simulink model "afc_simulation"  (R2019a)
settings: Solver=FixedStepDiscrete  StartTime=0.0  StopTime=50  RelTol=1e-3  EnableMultiTasking=on
values from neighbouring files (symbols this model uses):
  Cbus = 4*P/Vdc_min^2/4/fg    (= 0.0136971290817)    [afc_param.m]
  Cbus_2 = Cbus*2    (= 0.0273942581635)    [afc_param.m]
  Lf_1 = L1    [afc_param.m]
  Lf_2 = L1    [afc_param.m]
  RLf_1 = Lf_1*25    [afc_param.m]
  RLf_2 = Lf_2*25    [afc_param.m]
  Tss = 10e-6    (= 1e-05)    [afc_param.m]
undefined symbols (not defined in the file or in its folder): Ion, Lithium
libraries: simulink x21, powerlib_meascontrol x21, powerlib x17, electricdrivelib x3
(part 1 of 2)
settings Model: Creator=c477  LastModifiedBy=c477
settings SolverCC: AutoInsertRateTranBlk=on
settings OptimizationCC: DefaultParameterBehavior=Inlined  UseDivisionForNetSlopeComputation=on  GainParamInheritBuiltInType=on  UseFloatMulNetSlope=on  InlineInvariantSignals=on  PassReuseOutputArgsAs=Individual arguments  ZeroExternalMemoryAtStartup=off  ZeroInternalMemoryAtStartup=off  NoFixptDivByZeroProtection=on  EfficientFloat2IntCast=on  LifeSpan=1  OptimizeBlockOrder=speed  DifferentSizesBufferReuse=on
settings DebuggingCC: ParameterTunabilityLossMsg=error
settings HardwareCC: ProdLongLongMode=on
settings SFSimCC: MATLABDynamicMemAlloc=off
settings RTWCC: SystemTargetFile=ert.tlc  TemplateMakefile=ert_default_tmf  GenerateReport=on  IncludeHyperlinkInReport=on  LaunchReport=on  TargetLang=C++  GenerateTraceInfo=on  GenerateTraceReport=on  GenerateTraceReportSl=on  GenerateTraceReportSf=on  GenerateTraceReportEml=on
settings CodeAppCC: ForceParamTrailComments=on  IgnoreCustomStorageClasses=off  OperatorAnnotations=on  SimulinkDataObjDesc=on  SFDataObjDesc=on  CustomSymbolStrGlobalVar=rt$N$M  CustomSymbolStrType=$N$M  CustomSymbolStrFcn=$N$M$F  CustomSymbolStrMacro=$N$M  InsertBlockDesc=on
settings ERTTargetCC: TargetLangStandard=C++03 (ISO)  GenerateSampleERTMain=on  IncludeMdlTerminateFcn=off  CombineSignalStateStructs=on  MultiInstanceERTCode=on  CodeInterfacePackaging=C++ class  SupportNonInlinedSFcns=on  InlinedParameterPlacement=NonHierarchical  RootIOFormat=Structure reference  ERTCustomFileTemplate=example_file_process.tlc  ERTFilePackagingFormat=CompactWithDataFile

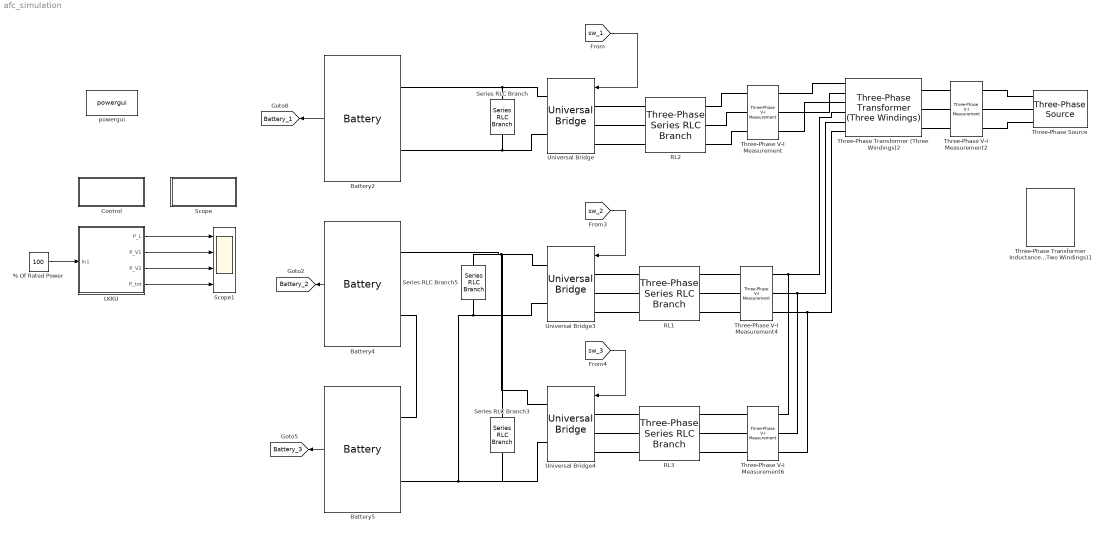
== system afc_simulation ==
  % Of Rated Power : Constant  Value=100
  Battery2 : electricdrivelib/Extra Sources/Battery  BatType=Lithium-Ion  ShowTempParam=off  ThermalPreset="3.3V  2.3Ah  (LiFePO4)"  ShowAgeParam=off  NomV=1000  NomQ=760  SOC=45  Batt_Tr=1  PresetModel=off  MaxQ=760  MinV=818  FullV=1082  Dis_rate=760  R=0.013158  Normal_OP=687.3043  expZone="[1080.3859       37.33913]"  current=[330.4348 330.4348*2 330.4348*5]  Units=Ampere-hour  Tci=20  NomT=25  T2=0  MaxQ2=2.208  FullV2=3.45  Normal_OP2=2.85  expZone2="[3.22       0.015]"  Rca=0.6  ti=1000  Dp=0  Neq0=0  Tsim=1e6  Ta1=25  Qeol=5.4*0.9  Reol=0.013333*1.2  Char_age=[2.3478, 3]  Dis_age=[2.3478, 10]  N1=1500  N2=10500  N3=1000  N4=1400  Ta2=45  N5=950
      settings: SourceProductName=Simscape Electrical
  Battery4 : electricdrivelib/Extra Sources/Battery  BatType=Lithium-Ion  ShowTempParam=off  ThermalPreset="3.3V  2.3Ah  (LiFePO4)"  ShowAgeParam=off  NomV=390  NomQ=641.0256  SOC=45  Batt_Tr=1  PresetModel=on  MaxQ=641.0256  MinV=292.5  FullV=453.955  Dis_rate=278.7068  R=0.006084  Normal_OP=579.7101  expZone="[421.3505      31.49387]"  current=[641.0256 641.0256*2 641.0256*5]  Units=Time  Tci=20  NomT=25  T2=0  MaxQ2=2.208  FullV2=3.45  Normal_OP2=2.85  expZone2="[3.22       0.015]"  Rca=0.6  ti=1000  Dp=0  Neq0=0  Tsim=1e6  Ta1=25  Qeol=5.4*0.9  Reol=0.013333*1.2  Char_age=[2.3478, 3]  Dis_age=[2.3478, 10]  N1=1500  N2=10500  N3=1000  N4=1400  Ta2=45  N5=950
      settings: SourceProductName=Simscape Electrical
  Battery5 : electricdrivelib/Extra Sources/Battery  BatType=Lithium-Ion  ShowTempParam=off  ThermalPreset="3.3V  2.3Ah  (LiFePO4)"  ShowAgeParam=off  NomV=390*2  NomQ=641.0256  SOC=45  Batt_Tr=1  PresetModel=on  MaxQ=641.0256  MinV=585  FullV=907.91  Dis_rate=278.7068  R=0.012168  Normal_OP=579.7101  expZone="[842.701      31.49387]"  current=[641.0256 641.0256*2 641.0256*5]  Units=Time  Tci=20  NomT=25  T2=0  MaxQ2=2.208  FullV2=3.45  Normal_OP2=2.85  expZone2="[3.22       0.015]"  Rca=0.6  ti=1000  Dp=0  Neq0=0  Tsim=1e6  Ta1=25  Qeol=5.4*0.9  Reol=0.013333*1.2  Char_age=[2.3478, 3]  Dis_age=[2.3478, 10]  N1=1500  N2=10500  N3=1000  N4=1400  Ta2=45  N5=950
      settings: SourceProductName=Simscape Electrical
  Control : Subsystem
  LKKU : Subsystem
  RL1 : powerlib/Elements/Three-Phase Series RLC Branch  LConnTagsString=A|B|C  RConnTagsString=A|B|C  BranchType=RL  Resistance=RLf_2  Inductance=Lf_2*1.3  Capacitance=1e-6  Measurements=None
      settings: SourceProductName=Simscape Electrical
  RL2 : powerlib/Elements/Three-Phase Series RLC Branch  LConnTagsString=A|B|C  RConnTagsString=A|B|C  BranchType=RL  Resistance=RLf_1  Inductance=Lf_1  Capacitance=1e-6  Measurements=None
      settings: SourceProductName=Simscape Electrical
  RL3 : powerlib/Elements/Three-Phase Series RLC Branch  LConnTagsString=A|B|C  RConnTagsString=A|B|C  BranchType=RL  Resistance=RLf_2  Inductance=Lf_2*1.3  Capacitance=1e-6  Measurements=None
      settings: SourceProductName=Simscape Electrical
  Scope : Subsystem
  Scope1 : Scope  NumInputPorts=4
  Series RLC Branch : powerlib/Elements/Series RLC Branch  LConnTagsString=__new0  RConnTagsString=__new0  BranchType=C  Resistance=1e-3  Inductance=1e-3  SetiL0=off  InitialCurrent=0  Capacitance=Cbus  Setx0=off  InitialVoltage=0  Measurements=None
      settings: SourceProductName=Simscape Electrical
  Series RLC Branch3 : powerlib/Elements/Series RLC Branch  LConnTagsString=__new0  RConnTagsString=__new0  BranchType=C  Resistance=1e-3  Inductance=1e-3  SetiL0=off  InitialCurrent=0  Capacitance=Cbus_2  Setx0=off  InitialVoltage=0  Measurements=None
      settings: SourceProductName=Simscape Electrical
  Series RLC Branch5 : powerlib/Elements/Series RLC Branch  LConnTagsString=__new0  RConnTagsString=__new0  BranchType=C  Resistance=1e-3  Inductance=1e-3  SetiL0=off  InitialCurrent=0  Capacitance=Cbus_2  Setx0=off  InitialVoltage=0  Measurements=None
      settings: SourceProductName=Simscape Electrical
  Three-Phase Transformer (Three Windings)2 : powerlib/Elements/Three-Phase Transformer (Three Windings)  Winding1Connection=Yg  Winding2Connection=Yg  Winding3Connection=Yg  CoreType=Three single-phase transformers  SetSaturation=off  Hysteresis=off  DataFile='hysteresis'  SetInitialFlux=off  Measurements=None  UNITS=pu  NominalPower=[ 2.5e6 , 60 ]  Winding1=[ 22.8e3, 0, 0]  Winding2=[ 550, 0 , 0]  Winding3=[ 380 , 0 , 0]  Rm=500  Lm=500  L0=0.5  Saturation=[ 0,0 ; 0.0024,1.2 ; 1.0,1.52 ]  InitialFluxes=[0.8 -0.8 0.7]  BreakLoop=on  DiscreteSolver=Trapezoidal iterative  DataType=off  TransfoNumber=1
      settings: SourceProductName=Simscape Electrical  SourceProductBaseCode=PS
  Three-Phase V-I Measurement : powerlib/Measurements/Three-Phase V-I Measurement  VoltageMeasurement=phase-to-ground  SetLabelV=on  LabelV=Vabc_1  Vpu=off  VpuLL=off  CurrentMeasurement=yes  SetLabelI=on  LabelI=Iabc_1  Ipu=off  Pbase=100e6  Vbase=500e3  OutputType=Complex  PhasorSimulation=off  PSBequivalent=0
      settings: SourceProductName=Simscape Electrical
  Three-Phase V-I Measurement2 : powerlib/Measurements/Three-Phase V-I Measurement  VoltageMeasurement=phase-to-ground  SetLabelV=on  LabelV=Vgrid  Vpu=off  VpuLL=off  CurrentMeasurement=yes  SetLabelI=on  LabelI=Igrid  Ipu=off  Pbase=100e6  Vbase=500e3  OutputType=Complex  PhasorSimulation=off  PSBequivalent=0
      settings: SourceProductName=Simscape Electrical
  Three-Phase V-I Measurement4 : powerlib/Measurements/Three-Phase V-I Measurement  VoltageMeasurement=phase-to-ground  SetLabelV=on  LabelV=Vabc_2  Vpu=off  VpuLL=off  CurrentMeasurement=yes  SetLabelI=on  LabelI=Iabc_2  Ipu=off  Pbase=100e6  Vbase=500e3  OutputType=Complex  PhasorSimulation=off  PSBequivalent=0
      settings: SourceProductName=Simscape Electrical
  Three-Phase V-I Measurement6 : powerlib/Measurements/Three-Phase V-I Measurement  VoltageMeasurement=phase-to-ground  SetLabelV=on  LabelV=Vabc_3  Vpu=off  VpuLL=off  CurrentMeasurement=yes  SetLabelI=on  LabelI=Iabc_3  Ipu=off  Pbase=100e6  Vbase=500e3  OutputType=Complex  PhasorSimulation=off  PSBequivalent=0
      settings: SourceProductName=Simscape Electrical
  Three-Phase Source : powerlib/Electrical Sources/Three-Phase Source  InternalConnection=Yg  VoltagePhases=off  Voltage=22.8e3  PhaseAngle=0  Voltage_phases=[25e3 25e3 25e3]/sqrt(3)  PhaseAngles_phases=[0 -120 +120]  Frequency=60  NonIdealSource=off  SpecifyImpedance=off  Resistance=0.8929  Inductance=16.58e-3  ShortCircuitLevel=100e6  BaseVoltage=25e3  XRratio=7  BusType=swing  Pref=10e3  Qref=0  Prefabc=[10e3, 10e3, 10e3]  Qrefabc=[0, 0, 0]  Qmin=-inf  Qmax=inf
      settings: SourceProductName=Simscape Electrical
  Three-Phase Transformer Inductance Matrix Type (Two Windings)1 : powerlib/Elements/Three-Phase Transformer Inductance Matrix Type (Two Windings)  CoreType=Three-limb or five-limb core  Winding1Connection=Yg  Winding2Connection=Yg  AutoTransformer=off  Measurements=None  NominalPower=[1e6, 60]  VLLnom=[22.8e3, 550]  WindingResistances=[0, 0]  NoLoadIexcPos=2  NoLoadPlossPos=1000  ShortCircuitReactancePos=0.06  ShortCircuitReactancePosAuto=0.06  NoLoadIexcZero=100  NoLoadPlossZero=1500  ShortCircuitReactanceZero=0.03  ShortCircuitReactanceZeroAuto=0.03
      settings: SourceProductName=Simscape Electrical  SourceProductBaseCode=PS
  Universal Bridge : powerlib/Power Electronics/Universal Bridge  Arms=3  SnubberResistance=1e5  SnubberCapacitance=inf  Device=IGBT / Diodes  Ron=1e-3  Lon=0  ForwardVoltages="[  0  0  ]"  ForwardVoltage=0  GTOparameters=[ 10e-6 , 20e-6 ]  IGBTparameters=[ 1e-6 , 2e-6 ]  Measurements=None  Measurements_2=None  converterType=Rectifier
      settings: SourceProductName=Simscape Electrical
  Universal Bridge3 : powerlib/Power Electronics/Universal Bridge  Arms=3  SnubberResistance=1e5  SnubberCapacitance=inf  Device=IGBT / Diodes  Ron=1e-3  Lon=0  ForwardVoltages="[  0  0  ]"  ForwardVoltage=0  GTOparameters=[ 10e-6 , 20e-6 ]  IGBTparameters=[ 1e-6 , 2e-6 ]  Measurements=None  Measurements_2=None  converterType=Rectifier
      settings: SourceProductName=Simscape Electrical
  Universal Bridge4 : powerlib/Power Electronics/Universal Bridge  Arms=3  SnubberResistance=1e5  SnubberCapacitance=inf  Device=IGBT / Diodes  Ron=1e-3  Lon=0  ForwardVoltages="[  0  0  ]"  ForwardVoltage=0  GTOparameters=[ 10e-6 , 20e-6 ]  IGBTparameters=[ 1e-6 , 2e-6 ]  Measurements=None  Measurements_2=None  converterType=Rectifier
      settings: SourceProductName=Simscape Electrical
  powergui : powerlib/powergui  Priority=1  SimulationMode=Discrete  SampleTime=Tss  frequency=60  Iterations=50  frequencyindice=0  Pbase=100e6  ErrMax=1e-4  UnitsV=kV  UnitsW=MW  buscounter=0  FunctionMessages=off  echomessages=off  EnableUseOfTLC=off  CurrentSourceSwitches=off  DisableSnubberDevices=off  DisableRonSwitches=off  DisableVfSwitches=off  DisplayEquations=off  AutomaticDiscreteSolvers=off  SolverType=Tustin/Backward Euler (TBE)  Interpol=off  ExternalGateDelay=off  methode=off  Ts=100  x0status=blocks  SPID=on  SwTol=0  HookPort=off  NonlinearTolerance=0  nMaxIteration=15  ContinueOnMaxIteration=off  RestoreLinks=warning  ResistiveCurrentMeasurement=off  Frange=[0:2:500]  Ylog=off  Xlog=on  ShowGrid=off  save=off  variable=ZData  structure=0  ZoomFFT=off  StartTime=0.0  cycles=1  DisplayStyle=1  fundamental=60  FreqAxis=off  MaxFrequency=1000  frequencyindicesteady=1  RmsSteady=1  display=off
      settings: SourceProductName=Simscape Electrical
  tag scope: Battery_1=global, Battery_2=global, Battery_3=global
  wires:
  Battery2/1 -> [Battery_1]
  [sw_1] -> Universal Bridge/1
  [sw_2] -> Universal Bridge3/1
  Battery4/1 -> [Battery_2]
  Battery5/1 -> [Battery_3]
  [sw_3] -> Universal Bridge4/1
  % Of Rated Power/1 -> LKKU/1(In1)
  LKKU/1(P_L) -> Scope1/1
  LKKU/2(P_V1) -> Scope1/2
  LKKU/3(P_V2) -> Scope1/3
  LKKU/4(P_tot) -> Scope1/4
  connections:
  RL2/LConn2 -- Universal Bridge/LConn2
  RL2/LConn1 -- Universal Bridge/LConn1
  RL2/LConn3 -- Universal Bridge/LConn3
  Universal Bridge/RConn2 -- Series RLC Branch/RConn1 -- Battery2/LConn2
  Universal Bridge/RConn1 -- Series RLC Branch/LConn1 -- Battery2/LConn1
  Three-Phase Source/RConn1 -- Three-Phase V-I Measurement2/LConn1
  Three-Phase V-I Measurement2/LConn2 -- Three-Phase Source/RConn2
  Three-Phase V-I Measurement2/LConn3 -- Three-Phase Source/RConn3
  Three-Phase V-I Measurement/LConn3 -- RL2/RConn3
  Three-Phase V-I Measurement/LConn1 -- RL2/RConn1
  Three-Phase V-I Measurement/LConn2 -- RL2/RConn2
  Three-Phase V-I Measurement6/RConn1 -- Three-Phase V-I Measurement4/RConn1 -- Three-Phase Transformer (Three Windings)2/RConn4
  Three-Phase V-I Measurement6/RConn2 -- Three-Phase Transformer (Three Windings)2/RConn5 -- Three-Phase V-I Measurement4/RConn2
  Three-Phase V-I Measurement6/RConn3 -- Three-Phase Transformer (Three Windings)2/RConn6 -- Three-Phase V-I Measurement4/RConn3
  Battery4/LConn2 -- Battery5/LConn1
  RL1/LConn1 -- Universal Bridge3/LConn1
  RL1/LConn2 -- Universal Bridge3/LConn2
  RL1/LConn3 -- Universal Bridge3/LConn3
  RL1/RConn2 -- Three-Phase V-I Measurement4/LConn2
  RL1/RConn1 -- Three-Phase V-I Measurement4/LConn1
  RL1/RConn3 -- Three-Phase V-I Measurement4/LConn3
  Universal Bridge3/RConn1 -- Series RLC Branch5/LConn1 -- Battery4/LConn1 -- Universal Bridge4/RConn1 -- Series RLC Branch3/LConn1
  RL3/RConn1 -- Three-Phase V-I Measurement6/LConn1
  RL3/LConn3 -- Universal Bridge4/LConn3
  RL3/LConn2 -- Universal Bridge4/LConn2
  RL3/LConn1 -- Universal Bridge4/LConn1
  RL3/RConn2 -- Three-Phase V-I Measurement6/LConn2
  RL3/RConn3 -- Three-Phase V-I Measurement6/LConn3
  Series RLC Branch5/RConn1 -- Universal Bridge3/RConn2 -- Universal Bridge4/RConn2 -- Series RLC Branch3/RConn1 -- Battery5/LConn2
  Three-Phase Transformer (Three Windings)2/LConn1 -- Three-Phase V-I Measurement2/RConn1
  Three-Phase Transformer (Three Windings)2/LConn2 -- Three-Phase V-I Measurement2/RConn2
  Three-Phase Transformer (Three Windings)2/LConn3 -- Three-Phase V-I Measurement2/RConn3
  Three-Phase Transformer (Three Windings)2/RConn1 -- Three-Phase V-I Measurement/RConn1
  Three-Phase Transformer (Three Windings)2/RConn2 -- Three-Phase V-I Measurement/RConn2
  Three-Phase Transformer (Three Windings)2/RConn3 -- Three-Phase V-I Measurement/RConn3

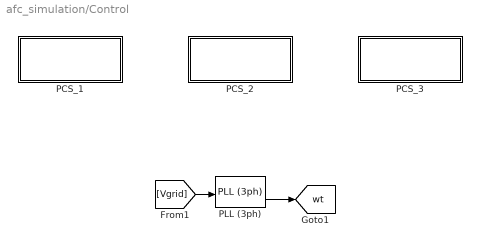
== system afc_simulation/Control ==
  PCS_1 : Subsystem
  PCS_2 : Subsystem
  PCS_3 : Subsystem
  PLL (3ph) : powerlib_meascontrol/PLL/PLL (3ph)  Fmin=45  Par_Init=[0, 50]  ParK=[180, 3200, 1]  TcD=1e-4  MaxRateChangeFreq=12  FilterCutOffFreq=25  Ts=Tss  AGC=on
      settings: SourceProductName=Simscape Electrical
  tag scope: wt=global
  wires:
  [Vgrid] -> PLL (3ph)/1
  PLL (3ph)/2 -> [wt]

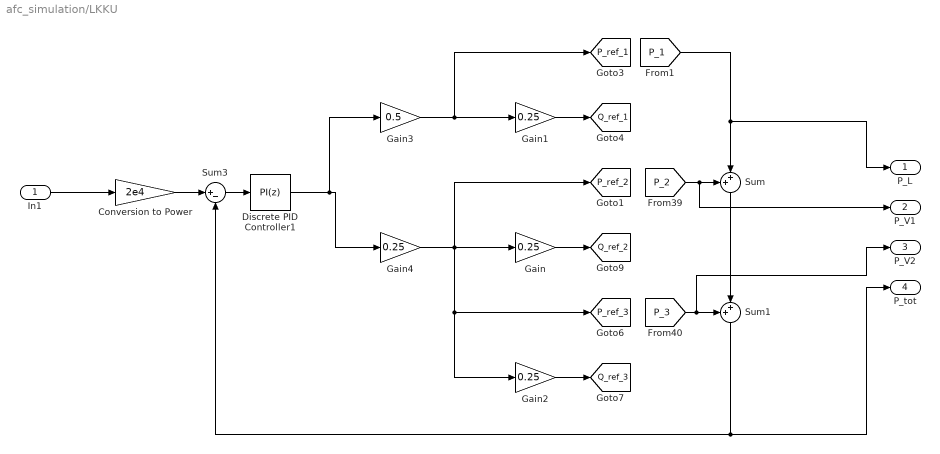
== system afc_simulation/LKKU ==
  In1 : Inport
  Conversion to Power : Gain  Gain=2e4
  Discrete PID Controller1 : simulink/Continuous/PID Controller  Controller=PI  Form=Parallel  TimeDomain=Discrete-time  SampleTime=Tss*30  IntegratorMethod=Forward Euler  FilterMethod=Forward Euler  ControllerParametersSource=internal  P=30  I=60  D=0.5  UseFilter=on  N=100  TunerSelectOption=Transfer Function Based (PID Tuner App)  InitialConditionSource=internal  InitialConditionForIntegrator=0  InitialConditionForFilter=0  DifferentiatorICPrevScaledInput=0  ExternalReset=none  TrackingMode=off  Kt=1  LimitOutput=off  UpperSaturationLimit=inf  LowerSaturationLimit=-inf  LinearizeAsGain=off  AntiWindupMode=none  Kb=1  POutMin=[]  POutMax=[]  IOutMin=[]  IOutMax=[]  DOutMin=[]  DOutMax=[]  NOutMin=[]  NOutMax=[]  SumOutMin=[]  SumOutMax=[]  SaturationOutMin=[]  SaturationOutMax=[]  PParamMin=[]  PParamMax=[]  IParamMin=[]  IParamMax=[]  DParamMin=[]  DParamMax=[]  NParamMin=[]  NParamMax=[]  KbParamMin=[]  KbParamMax=[]  KtParamMin=[]  KtParamMax=[]  KbOutMin=[]  KbOutMax=[]  KtOutMin=[]  KtOutMax=[]  IntegratorOutMin=[]  IntegratorOutMax=[]  FilterOutMin=[]  FilterOutMax=[]  SumI1OutMin=[]  SumI1OutMax=[]  SumI2OutMin=[]  SumI2OutMax=[]  SumI3OutMin=[]  SumI3OutMax=[]  SumI4OutMin=[]  SumI4OutMax=[]  SumDOutMin=[]  SumDOutMax=[]  DifferentiatorOutMin=[]  DifferentiatorOutMax=[]  FilterDiffOutCoefMin=[]  FilterDiffOutCoefMax=[]  ReciprocalOutMin=[]  ReciprocalOutMax=[]  SumDenOutMin=[]  SumDenOutMax=[]  SumNumOutMin=[]  SumNumOutMax=[]  DivideOutMin=[]  DivideOutMax=[]  IntegratorContinuousStateAttributes=''  IntegratorStateMustResolveToSignalObject=off  IntegratorRTWStateStorageClass=Auto  FilterContinuousStateAttributes=''  FilterStateMustResolveToSignalObject=off  FilterRTWStateStorageClass=Auto  ParallelPVariant=InternalParameters  IdealPVariant=Disabled  IVariant=InternalParameters  DVariant=Disabled  IntegratorVariant=Discrete  SatVariant=Disabled  AWVariant=Passthrough  PCopyVariant=Disabled  TRVariant=Disabled  FdbkBlocksVariant=Forward  IdealPFdbkVariant=Disabled  SatFdbkVariant=Disabled  DerivativeFilterVariant=Disabled  NVariant=Disabled  NCopyVariant=Disabled_SignalSpec  FilterICVariant=Disabled  IntegratorICVariant=InternalICs  ExternalResetVariant=Disabled  TRSumVariant=Passthrough  SumFdbkVariant=Disabled  SumVariant=Sum_PI
  Gain{,1..2,4} (4 alike) : Gain  Gain=0.25
  Gain3 : Gain  Gain=0.5
  Sum : Sum  Inputs=++|
  Sum1 : Sum  Inputs=++|
  Sum3 : Sum  Inputs=|+-
  P_L : Outport
  P_V1 : Outport  Port=2
  P_V2 : Outport  Port=3
  P_tot : Outport  Port=4
  tag scope: P_ref_1=global, P_ref_2=global, P_ref_3=global, Q_ref_1=global, Q_ref_2=global, Q_ref_3=global
  wires:
  Sum1/1 -> P_tot/1, Sum3/2
  In1/1 -> Conversion to Power/1
  [P_2] -> P_V1/1, Sum/1
  Discrete PID Controller1/1 -> Gain3/1, Gain4/1
  [P_3] -> P_V2/1, Sum1/1
  Conversion to Power/1 -> Sum3/1
  Gain4/1 -> [P_ref_3], Gain2/1, [P_ref_2], Gain/1
  Sum3/1 -> Discrete PID Controller1/1
  Sum/1 -> Sum1/2
  Gain1/1 -> [Q_ref_1]
  Gain2/1 -> [Q_ref_3]
  [P_1] -> P_L/1, Sum/2
  Gain3/1 -> [P_ref_1], Gain1/1
  Gain/1 -> [Q_ref_2]

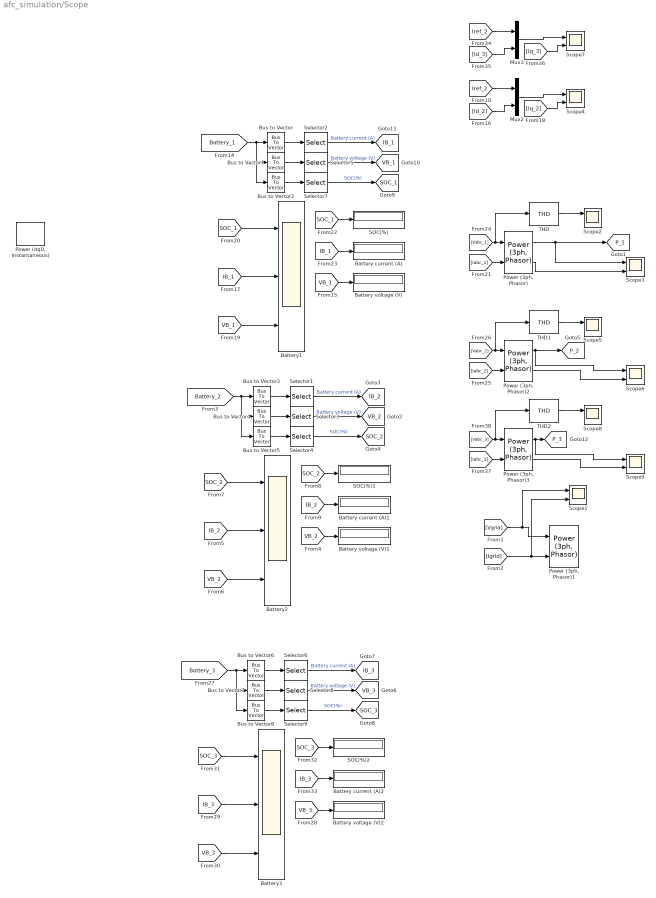
== system afc_simulation/Scope ==
  Battery current (A) : Display
  Battery current (A)1 : Display
  Battery current (A)2 : Display
  Battery voltage (V) : Display
  Battery voltage (V)1 : Display
  Battery voltage (V)2 : Display
  Battery1 : Scope  NumInputPorts=3
  Battery2 : Scope  NumInputPorts=3
  Battery3 : Scope  NumInputPorts=3
  Bus to Vector{,1..8} (9 alike) : BusToVector
  Mux2 : Mux  Inputs=2
  Mux3 : Mux  Inputs=2
  Power (3ph, Phasor){,1..3} (4 alike) : powerlib_meascontrol/Measurements/Power (3ph, Phasor)
      settings: SourceProductName=Simscape Electrical  SourceProductBaseCode=PS
  "Power (dq0, Instantaneous)" : powerlib_meascontrol/Measurements/Power (dq0, Instantaneous)
      settings: SourceProductName=Simscape Electrical  SourceProductBaseCode=PS
  SOC(%) : Display
  SOC(%)1 : Display
  SOC(%)2 : Display
  Scope{1..9} (9 alike) : Scope  NumInputPorts=2
  Selector1 : Selector  InputPortWidth=3  IndexOptions=Index vector (dialog)  Indices=[2]  OutputSizes=1
  Selector2 : Selector  InputPortWidth=3  IndexOptions=Index vector (dialog)  Indices=[2]  OutputSizes=1
  Selector3 : Selector  InputPortWidth=3  IndexOptions=Index vector (dialog)  Indices=[3]  OutputSizes=1
  Selector4 : Selector  InputPortWidth=3  IndexOptions=Index vector (dialog)  Indices=[1]  OutputSizes=1
  Selector5 : Selector  InputPortWidth=3  IndexOptions=Index vector (dialog)  Indices=[3]  OutputSizes=1
  Selector6 : Selector  InputPortWidth=3  IndexOptions=Index vector (dialog)  Indices=[2]  OutputSizes=1
  Selector7 : Selector  InputPortWidth=3  IndexOptions=Index vector (dialog)  Indices=[1]  OutputSizes=1
  Selector8 : Selector  InputPortWidth=3  IndexOptions=Index vector (dialog)  Indices=[3]  OutputSizes=1
  Selector9 : Selector  InputPortWidth=3  IndexOptions=Index vector (dialog)  Indices=[1]  OutputSizes=1
  THD : powerlib_meascontrol/Measurements/THD  Freq=60  Ts=Tss
      settings: SourceProductName=Simscape Electrical
  THD1 : powerlib_meascontrol/Measurements/THD  Freq=60  Ts=Tss
      settings: SourceProductName=Simscape Electrical
  THD2 : powerlib_meascontrol/Measurements/THD  Freq=60  Ts=Tss
      settings: SourceProductName=Simscape Electrical
  tag scope: IB_1=global, IB_2=global, IB_3=global, P_1=global, P_2=global, P_3=global, SOC_1=global, SOC_2=global, SOC_3=global, VB_1=global, VB_2=global, VB_3=global
  wires:
  [IB_1] -> Battery current (A)/1
  Selector7/1 -> [SOC_1]  "SOC(%)"
  Bus to Vector1/1 -> Selector5/1
  [VB_1] -> Battery1/3
  [VB_1] -> Battery voltage (V)/1
  [SOC_1] -> Battery1/1
  [SOC_1] -> SOC(%)/1
  Selector2/1 -> [IB_1]  "Battery current (A)"
  Bus to Vector/1 -> Selector2/1
  [IB_1] -> Battery1/2
  Selector5/1 -> [VB_1]  "Battery voltage (V)"
  Bus to Vector2/1 -> Selector7/1
  [Battery_1] -> Bus to Vector/1, Bus to Vector1/1, Bus to Vector2/1
  [Vabc_1] -> THD/1, "Power (3ph, Phasor)"/1
  [Iabc_1] -> "Power (3ph, Phasor)"/2
  "Power (3ph, Phasor)"/2 -> Scope3/2
  [Vgrid] -> Scope1/1, "Power (3ph, Phasor)1"/1
  [Igrid] -> Scope1/2, "Power (3ph, Phasor)1"/2
  THD/1 -> Scope2/1
  [Battery_2] -> Bus to Vector5/1, Bus to Vector4/1, Bus to Vector3/1
  Bus to Vector5/1 -> Selector4/1
  Selector3/1 -> [VB_2]  "Battery voltage (V)"
  [IB_2] -> Battery2/2
  Bus to Vector3/1 -> Selector1/1
  Selector1/1 -> [IB_2]  "Battery current (A)"
  [SOC_2] -> SOC(%)1/1
  [SOC_2] -> Battery2/1
  [VB_2] -> Battery voltage (V)1/1
  [VB_2] -> Battery2/3
  Bus to Vector4/1 -> Selector3/1
  Selector4/1 -> [SOC_2]  "SOC(%)"
  [IB_2] -> Battery current (A)1/1
  [Iref_2] -> Mux2/1
  [Iq_2] -> Scope4/2
  Mux2/1 -> Scope4/1
  [Id_2] -> Mux2/2
  THD1/1 -> Scope5/1
  "Power (3ph, Phasor)2"/1 -> [P_2], Scope6/1
  "Power (3ph, Phasor)2"/2 -> Scope6/2
  [Iabc_2] -> "Power (3ph, Phasor)2"/2
  [Vabc_2] -> "Power (3ph, Phasor)2"/1, THD1/1
  [IB_3] -> Battery current (A)2/1
  Selector9/1 -> [SOC_3]  "SOC(%)"
  Bus to Vector7/1 -> Selector8/1
  [VB_3] -> Battery3/3
  [VB_3] -> Battery voltage (V)2/1
  [SOC_3] -> Battery3/1
  [SOC_3] -> SOC(%)2/1
  Selector6/1 -> [IB_3]  "Battery current (A)"
  Bus to Vector6/1 -> Selector6/1
  [IB_3] -> Battery3/2
  Selector8/1 -> [VB_3]  "Battery voltage (V)"
  Bus to Vector8/1 -> Selector9/1
  [Battery_3] -> Bus to Vector6/1, Bus to Vector7/1, Bus to Vector8/1
  [Id_3] -> Mux3/2
  Mux3/1 -> Scope7/1
  [Iq_3] -> Scope7/2
  [Iref_2] -> Mux3/1
  [Vabc_3] -> THD2/1, "Power (3ph, Phasor)3"/1
  [Iabc_3] -> "Power (3ph, Phasor)3"/2
  "Power (3ph, Phasor)3"/2 -> Scope9/2
  "Power (3ph, Phasor)3"/1 -> Scope9/1, [P_3]
  THD2/1 -> Scope8/1
  "Power (3ph, Phasor)"/1 -> [P_1], Scope3/1

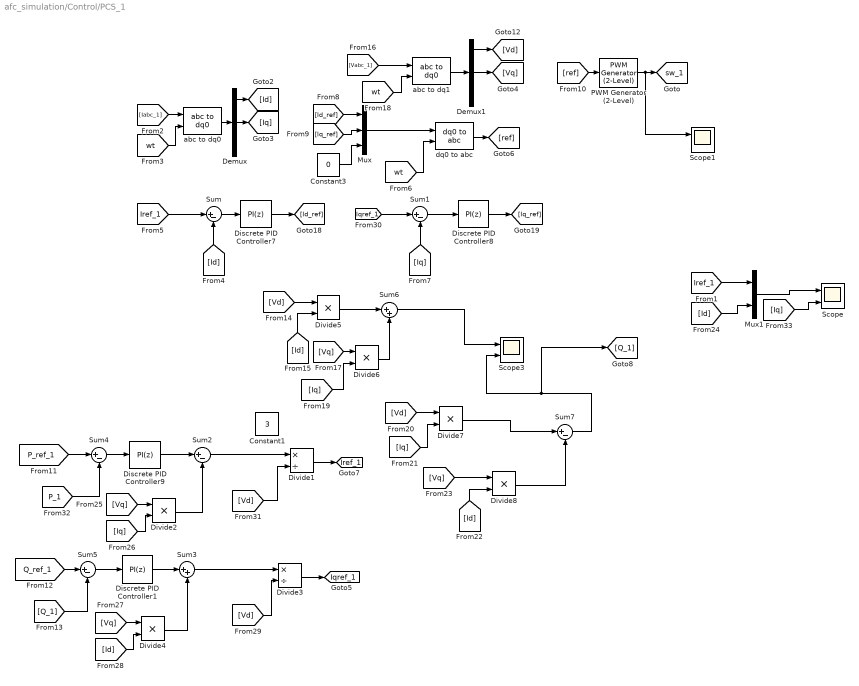
== system afc_simulation/Control/PCS_1 ==
  Constant1 : Constant  Value=3
  Constant3 : Constant  Value=0
  Demux : Demux  Outputs=3
  Demux1 : Demux  Outputs=3
  Discrete PID Controller1 : simulink/Continuous/PID Controller  Controller=PI  Form=Parallel  TimeDomain=Discrete-time  SampleTime=Tss  IntegratorMethod=Forward Euler  FilterMethod=Forward Euler  ControllerParametersSource=internal  P=0.001  I=10  D=0.0001  UseFilter=on  N=100  TunerSelectOption=Transfer Function Based (PID Tuner App)  InitialConditionSource=internal  InitialConditionForIntegrator=0  InitialConditionForFilter=0  DifferentiatorICPrevScaledInput=0  ExternalReset=none  TrackingMode=off  Kt=1  LimitOutput=off  UpperSaturationLimit=1.2  LowerSaturationLimit=0  LinearizeAsGain=off  AntiWindupMode=none  Kb=1  POutMin=[]  POutMax=[]  IOutMin=[]  IOutMax=[]  DOutMin=[]  DOutMax=[]  NOutMin=[]  NOutMax=[]  SumOutMin=[]  SumOutMax=[]  SaturationOutMin=[]  SaturationOutMax=[]  PParamMin=[]  PParamMax=[]  IParamMin=[]  IParamMax=[]  DParamMin=[]  DParamMax=[]  NParamMin=[]  NParamMax=[]  KbParamMin=[]  KbParamMax=[]  KtParamMin=[]  KtParamMax=[]  KbOutMin=[]  KbOutMax=[]  KtOutMin=[]  KtOutMax=[]  IntegratorOutMin=[]  IntegratorOutMax=[]  FilterOutMin=[]  FilterOutMax=[]  SumI1OutMin=[]  SumI1OutMax=[]  SumI2OutMin=[]  SumI2OutMax=[]  SumI3OutMin=[]  SumI3OutMax=[]  SumI4OutMin=[]  SumI4OutMax=[]  SumDOutMin=[]  SumDOutMax=[]  DifferentiatorOutMin=[]  DifferentiatorOutMax=[]  FilterDiffOutCoefMin=[]  FilterDiffOutCoefMax=[]  ReciprocalOutMin=[]  ReciprocalOutMax=[]  SumDenOutMin=[]  SumDenOutMax=[]  SumNumOutMin=[]  SumNumOutMax=[]  DivideOutMin=[]  DivideOutMax=[]  IntegratorContinuousStateAttributes=''  IntegratorStateMustResolveToSignalObject=off  IntegratorRTWStateStorageClass=Auto  FilterContinuousStateAttributes=''  FilterStateMustResolveToSignalObject=off  FilterRTWStateStorageClass=Auto  ParallelPVariant=InternalParameters  IdealPVariant=Disabled  IVariant=InternalParameters  DVariant=Disabled  IntegratorVariant=Discrete  SatVariant=Disabled  AWVariant=Passthrough  PCopyVariant=Disabled  TRVariant=Disabled  FdbkBlocksVariant=Forward  IdealPFdbkVariant=Disabled  SatFdbkVariant=Disabled  DerivativeFilterVariant=Disabled  NVariant=Disabled  NCopyVariant=Disabled_SignalSpec  FilterICVariant=Disabled  IntegratorICVariant=InternalICs  ExternalResetVariant=Disabled  TRSumVariant=Passthrough  SumFdbkVariant=Disabled  SumVariant=Sum_PI
  Discrete PID Controller7 : simulink/Continuous/PID Controller  Controller=PI  Form=Parallel  TimeDomain=Discrete-time  SampleTime=Tss  IntegratorMethod=Forward Euler  FilterMethod=Forward Euler  ControllerParametersSource=internal  P=2  I=3  D=0  UseFilter=on  N=100  TunerSelectOption=Transfer Function Based (PID Tuner App)  InitialConditionSource=internal  InitialConditionForIntegrator=0  InitialConditionForFilter=0  DifferentiatorICPrevScaledInput=0  ExternalReset=none  TrackingMode=off  Kt=1  LimitOutput=off  UpperSaturationLimit=1.2  LowerSaturationLimit=0  LinearizeAsGain=off  AntiWindupMode=none  Kb=1  POutMin=[]  POutMax=[]  IOutMin=[]  IOutMax=[]  DOutMin=[]  DOutMax=[]  NOutMin=[]  NOutMax=[]  SumOutMin=[]  SumOutMax=[]  SaturationOutMin=[]  SaturationOutMax=[]  PParamMin=[]  PParamMax=[]  IParamMin=[]  IParamMax=[]  DParamMin=[]  DParamMax=[]  NParamMin=[]  NParamMax=[]  KbParamMin=[]  KbParamMax=[]  KtParamMin=[]  KtParamMax=[]  KbOutMin=[]  KbOutMax=[]  KtOutMin=[]  KtOutMax=[]  IntegratorOutMin=[]  IntegratorOutMax=[]  FilterOutMin=[]  FilterOutMax=[]  SumI1OutMin=[]  SumI1OutMax=[]  SumI2OutMin=[]  SumI2OutMax=[]  SumI3OutMin=[]  SumI3OutMax=[]  SumI4OutMin=[]  SumI4OutMax=[]  SumDOutMin=[]  SumDOutMax=[]  DifferentiatorOutMin=[]  DifferentiatorOutMax=[]  FilterDiffOutCoefMin=[]  FilterDiffOutCoefMax=[]  ReciprocalOutMin=[]  ReciprocalOutMax=[]  SumDenOutMin=[]  SumDenOutMax=[]  SumNumOutMin=[]  SumNumOutMax=[]  DivideOutMin=[]  DivideOutMax=[]  IntegratorContinuousStateAttributes=''  IntegratorStateMustResolveToSignalObject=off  IntegratorRTWStateStorageClass=Auto  FilterContinuousStateAttributes=''  FilterStateMustResolveToSignalObject=off  FilterRTWStateStorageClass=Auto  ParallelPVariant=InternalParameters  IdealPVariant=Disabled  IVariant=InternalParameters  DVariant=Disabled  IntegratorVariant=Discrete  SatVariant=Disabled  AWVariant=Passthrough  PCopyVariant=Disabled  TRVariant=Disabled  FdbkBlocksVariant=Forward  IdealPFdbkVariant=Disabled  SatFdbkVariant=Disabled  DerivativeFilterVariant=Disabled  NVariant=Disabled  NCopyVariant=Disabled_SignalSpec  FilterICVariant=Disabled  IntegratorICVariant=InternalICs  ExternalResetVariant=Disabled  TRSumVariant=Passthrough  SumFdbkVariant=Disabled  SumVariant=Sum_PI
  Discrete PID Controller8 : simulink/Continuous/PID Controller  Controller=PI  Form=Parallel  TimeDomain=Discrete-time  SampleTime=Tss  IntegratorMethod=Forward Euler  FilterMethod=Forward Euler  ControllerParametersSource=internal  P=2  I=3  D=0  UseFilter=on  N=100  TunerSelectOption=Transfer Function Based (PID Tuner App)  InitialConditionSource=internal  InitialConditionForIntegrator=0  InitialConditionForFilter=0  DifferentiatorICPrevScaledInput=0  ExternalReset=none  TrackingMode=off  Kt=1  LimitOutput=off  UpperSaturationLimit=1.1  LowerSaturationLimit=-1.1  LinearizeAsGain=off  AntiWindupMode=none  Kb=1  POutMin=[]  POutMax=[]  IOutMin=[]  IOutMax=[]  DOutMin=[]  DOutMax=[]  NOutMin=[]  NOutMax=[]  SumOutMin=[]  SumOutMax=[]  SaturationOutMin=[]  SaturationOutMax=[]  PParamMin=[]  PParamMax=[]  IParamMin=[]  IParamMax=[]  DParamMin=[]  DParamMax=[]  NParamMin=[]  NParamMax=[]  KbParamMin=[]  KbParamMax=[]  KtParamMin=[]  KtParamMax=[]  KbOutMin=[]  KbOutMax=[]  KtOutMin=[]  KtOutMax=[]  IntegratorOutMin=[]  IntegratorOutMax=[]  FilterOutMin=[]  FilterOutMax=[]  SumI1OutMin=[]  SumI1OutMax=[]  SumI2OutMin=[]  SumI2OutMax=[]  SumI3OutMin=[]  SumI3OutMax=[]  SumI4OutMin=[]  SumI4OutMax=[]  SumDOutMin=[]  SumDOutMax=[]  DifferentiatorOutMin=[]  DifferentiatorOutMax=[]  FilterDiffOutCoefMin=[]  FilterDiffOutCoefMax=[]  ReciprocalOutMin=[]  ReciprocalOutMax=[]  SumDenOutMin=[]  SumDenOutMax=[]  SumNumOutMin=[]  SumNumOutMax=[]  DivideOutMin=[]  DivideOutMax=[]  IntegratorContinuousStateAttributes=''  IntegratorStateMustResolveToSignalObject=off  IntegratorRTWStateStorageClass=Auto  FilterContinuousStateAttributes=''  FilterStateMustResolveToSignalObject=off  FilterRTWStateStorageClass=Auto  ParallelPVariant=InternalParameters  IdealPVariant=Disabled  IVariant=InternalParameters  DVariant=Disabled  IntegratorVariant=Discrete  SatVariant=Disabled  AWVariant=Passthrough  PCopyVariant=Disabled  TRVariant=Disabled  FdbkBlocksVariant=Forward  IdealPFdbkVariant=Disabled  SatFdbkVariant=Disabled  DerivativeFilterVariant=Disabled  NVariant=Disabled  NCopyVariant=Disabled_SignalSpec  FilterICVariant=Disabled  IntegratorICVariant=InternalICs  ExternalResetVariant=Disabled  TRSumVariant=Passthrough  SumFdbkVariant=Disabled  SumVariant=Sum_PI
  Discrete PID Controller9 : simulink/Continuous/PID Controller  Controller=PI  Form=Parallel  TimeDomain=Discrete-time  SampleTime=Tss  IntegratorMethod=Forward Euler  FilterMethod=Forward Euler  ControllerParametersSource=internal  P=0.01  I=10  D=0.0001  UseFilter=on  N=100  TunerSelectOption=Transfer Function Based (PID Tuner App)  InitialConditionSource=internal  InitialConditionForIntegrator=0  InitialConditionForFilter=0  DifferentiatorICPrevScaledInput=0  ExternalReset=none  TrackingMode=off  Kt=1  LimitOutput=off  UpperSaturationLimit=1.2  LowerSaturationLimit=0  LinearizeAsGain=off  AntiWindupMode=none  Kb=1  POutMin=[]  POutMax=[]  IOutMin=[]  IOutMax=[]  DOutMin=[]  DOutMax=[]  NOutMin=[]  NOutMax=[]  SumOutMin=[]  SumOutMax=[]  SaturationOutMin=[]  SaturationOutMax=[]  PParamMin=[]  PParamMax=[]  IParamMin=[]  IParamMax=[]  DParamMin=[]  DParamMax=[]  NParamMin=[]  NParamMax=[]  KbParamMin=[]  KbParamMax=[]  KtParamMin=[]  KtParamMax=[]  KbOutMin=[]  KbOutMax=[]  KtOutMin=[]  KtOutMax=[]  IntegratorOutMin=[]  IntegratorOutMax=[]  FilterOutMin=[]  FilterOutMax=[]  SumI1OutMin=[]  SumI1OutMax=[]  SumI2OutMin=[]  SumI2OutMax=[]  SumI3OutMin=[]  SumI3OutMax=[]  SumI4OutMin=[]  SumI4OutMax=[]  SumDOutMin=[]  SumDOutMax=[]  DifferentiatorOutMin=[]  DifferentiatorOutMax=[]  FilterDiffOutCoefMin=[]  FilterDiffOutCoefMax=[]  ReciprocalOutMin=[]  ReciprocalOutMax=[]  SumDenOutMin=[]  SumDenOutMax=[]  SumNumOutMin=[]  SumNumOutMax=[]  DivideOutMin=[]  DivideOutMax=[]  IntegratorContinuousStateAttributes=''  IntegratorStateMustResolveToSignalObject=off  IntegratorRTWStateStorageClass=Auto  FilterContinuousStateAttributes=''  FilterStateMustResolveToSignalObject=off  FilterRTWStateStorageClass=Auto  ParallelPVariant=InternalParameters  IdealPVariant=Disabled  IVariant=InternalParameters  DVariant=Disabled  IntegratorVariant=Discrete  SatVariant=Disabled  AWVariant=Passthrough  PCopyVariant=Disabled  TRVariant=Disabled  FdbkBlocksVariant=Forward  IdealPFdbkVariant=Disabled  SatFdbkVariant=Disabled  DerivativeFilterVariant=Disabled  NVariant=Disabled  NCopyVariant=Disabled_SignalSpec  FilterICVariant=Disabled  IntegratorICVariant=InternalICs  ExternalResetVariant=Disabled  TRSumVariant=Passthrough  SumFdbkVariant=Disabled  SumVariant=Sum_PI
  Divide1 : Product  Inputs=*/
  Divide{2,4..8} (6 alike) : Product  Inputs=**
  Divide3 : Product  Inputs=*/
  Mux : Mux  Inputs=3
  Mux1 : Mux  Inputs=2
  PWM Generator (2-Level) : powerlib_meascontrol/Pulse & Signal Generators/PWM Generator (2-Level)  ModulatorType=Three-phase bridge (6 pulses)  ModulatorMode=Unsynchronized  Fc=fsw  Pc=90  nF=27  MinMax="[ -1  1 ]"  SamplingTechnique=Natural  ModulatingSignals=off  m=0.8  Freq=60  Phase=0  Ts=Tss  ShowCarrierOutport=off
  Scope : Scope  NumInputPorts=2
  Scope1 : Scope  NumInputPorts=2
  Scope3 : Scope  NumInputPorts=2
  Sum{,1..2,4..5,7} (6 alike) : Sum  Inputs=|+-
  Sum3 : Sum  Inputs=|++
  Sum6 : Sum  Inputs=|++
  abc to dq0 : powerlib_meascontrol/Transformations/abc to dq0  Alignment=90 degrees behind phase A axis
      settings: SourceProductName=Simscape Electrical
  abc to dq1 : powerlib_meascontrol/Transformations/abc to dq0  Alignment=90 degrees behind phase A axis
      settings: SourceProductName=Simscape Electrical
  dq0 to abc : powerlib_meascontrol/Transformations/dq0 to abc  Alignment=90 degrees behind phase A axis
      settings: SourceProductName=Simscape Electrical
  tag scope: Iqref_1=global, Iref_1=global, sw_1=global
  wires:
  [P_1] -> Sum4/2
  Divide5/1 -> Sum6/1
  Divide6/1 -> Sum6/2
  [Vd] -> Divide1/2
  Divide7/1 -> Sum7/1
  [Q_1] -> Sum5/2
  [Vq] -> Divide6/1
  Discrete PID Controller7/1 -> [Id_ref]
  Demux/2 -> [Iq]
  Divide3/1 -> [Iqref_1]
  abc to dq1/1 -> Demux1/1
  Divide8/1 -> Sum7/2
  [Iq] -> Divide6/2
  [Iq] -> Divide2/2
  Demux1/2 -> [Vq]
  [Iq] -> Divide7/2
  [Vd] -> Divide7/1
  Sum2/1 -> Divide1/1
  Sum5/1 -> Discrete PID Controller1/1
  [Id] -> Divide5/2
  dq0 to abc/1 -> [ref]
  [Vd] -> Divide5/1
  [Vq] -> Divide4/1
  [P_ref_1] -> Sum4/1
  [wt] -> dq0 to abc/2
  [wt] -> abc to dq0/2
  [Q_ref_1] -> Sum5/1
  [Vd] -> Divide3/2
  Constant3/1 -> Mux/3
  [Iabc_1] -> abc to dq0/1
  Sum3/1 -> Divide3/1
  [Id] -> Divide4/2
  Discrete PID Controller9/1 -> Sum2/1
  Discrete PID Controller1/1 -> Sum3/1
  Sum/1 -> Discrete PID Controller7/1
  Divide4/1 -> Sum3/2
  PWM Generator (2-Level)/1 -> Scope1/1, [sw_1]
  [Vq] -> Divide2/1
  Demux/1 -> [Id]
  Sum4/1 -> Discrete PID Controller9/1
  [Id_ref] -> Mux/1
  abc to dq0/1 -> Demux/1
  [Iq] -> Sum1/2
  Sum1/1 -> Discrete PID Controller8/1
  Discrete PID Controller8/1 -> [Iq_ref]
  Divide2/1 -> Sum2/2
  Mux/1 -> dq0 to abc/1
  [Iqref_1] -> Sum1/1
  [Vq] -> Divide8/1
  [wt] -> abc to dq1/2
  Demux1/1 -> [Vd]
  [Iq_ref] -> Mux/2
  Sum7/1 -> [Q_1], Scope3/2
  [ref] -> PWM Generator (2-Level)/1
  [Id] -> Divide8/2
  [Id] -> Sum/2
  [Vabc_1] -> abc to dq1/1
  [Iref_1] -> Sum/1
  Divide1/1 -> [Iref_1]
  [Id] -> Mux1/2
  [Iq] -> Scope/2
  [Iref_1] -> Mux1/1
  Mux1/1 -> Scope/1
  Sum6/1 -> Scope3/1
